simulink model "Project_1"  (R2021a)
settings: Solver=VariableStepAuto  StartTime=0.0  StopTime=15  MaxStep=0.01  RelTol=1e-3
settings Model: Creator=ZeynepDilanKılıç  LastModifiedBy=ZeynepDilanKılıç

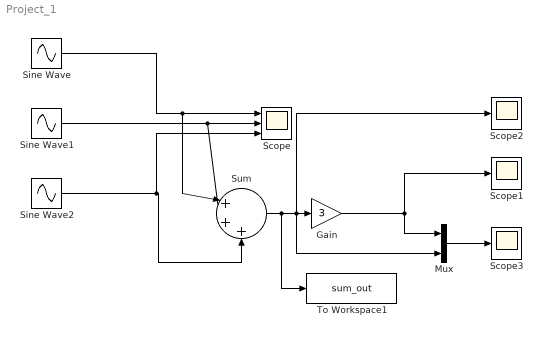
== system Project_1 ==
  Gain : Gain  Gain=3
  Mux : Mux  Inputs=2
  Scope : Scope  NumInputPorts=3
  Scope1 : Scope
  Scope2 : Scope
  Scope3 : Scope
  Sine Wave : Sin  SampleTime=0
  Sine Wave1 : Sin  Frequency=2  SampleTime=0
  Sine Wave2 : Sin  Frequency=10  SampleTime=0
  Sum : Sum  Inputs=|+++
  To Workspace1 : ToWorkspace  VariableName=sum_out  SaveFormat=Timeseries  SampleTime=-1
  wires:
  Sum/1 -> To Workspace1/1, Mux/2, Scope2/1, Gain/1
  Sine Wave/1 -> Sum/1, Scope/1
  Sine Wave1/1 -> Sum/2, Scope/2
  Sine Wave2/1 -> Sum/3, Scope/3
  Gain/1 -> Mux/1, Scope1/1
  Mux/1 -> Scope3/1
